simulink model "example"  (R2022a)
settings: Solver=VariableStepAuto  StartTime=0.0  StopTime=10.0  RelTol=1e-3
settings Model: Creator=ga53hon  LastModifiedBy=ga53hon

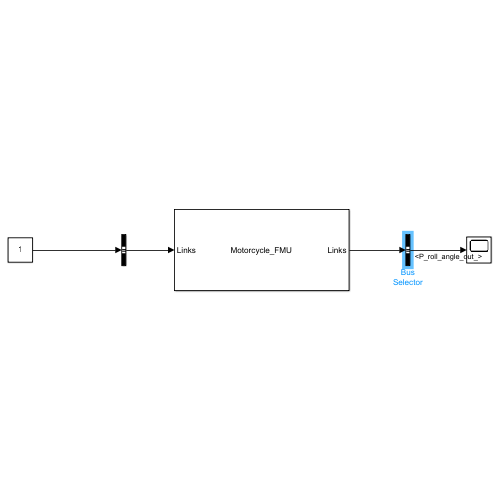
[thumbnail: Simulink's stored preview of the top-level diagram]
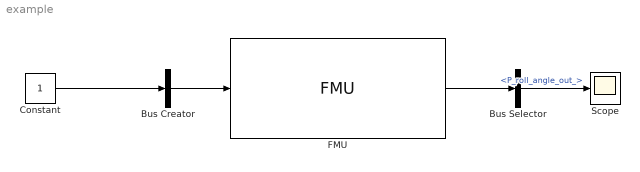
== system example ==
  Bus Creator : BusCreator  Inputs=1  OutDataTypeStr=Bus: mbs_in  NonVirtualBus=on
  Bus Selector : BusSelector  OutputSignals=P_roll_angle_out_
  Constant : Constant
  FMU : FMU  FMUName=mbsim.fmu  FMUMode=ModelExchange  P_Output_directory_=.  Plot=struct('mode',int32(2),'P_each_n_th_step_',int32(5),'P_sample_time_',0.001)  P_Constraint_tolerance_=struct('position',1.0000000000000001e-05,'velocity',1.0000000000000001e-05)  mask(Motorcycle_FMU [Model Exchange, v1.0]){}
      settings: MultithreadedSim=off
      mask Display:
      | disp('Motorcycle_FMU');
      | port_label('output',1,'Links');
      | port_label('input',1,'Links');
  Scope : Scope
  wires:
  Bus Creator/1 -> FMU/1
  Constant/1 -> Bus Creator/1
  FMU/1 -> Bus Selector/1
  Bus Selector/1 -> Scope/1  "<P_roll_angle_out_>"
